simulink model "gps_time_integrator_test"  (R2016b)
settings: Solver=VariableStepAuto  StartTime=0.0  StopTime=6000  RelTol=1e-3
values from neighbouring files (symbols this model uses):
  fsw_params = init_fsw_params()    [GPS_processing_test_init.m]
libraries: gps x1, GPS_processing_lib x1, GPS_time_lib x1, time_conversion_lib x1, MET_lib x1, time_coord_rotation_lib x1, tle2eci_coarse_lib x1
settings Model: Creator=taylorreynolds  LastModifiedBy=taylorreynolds

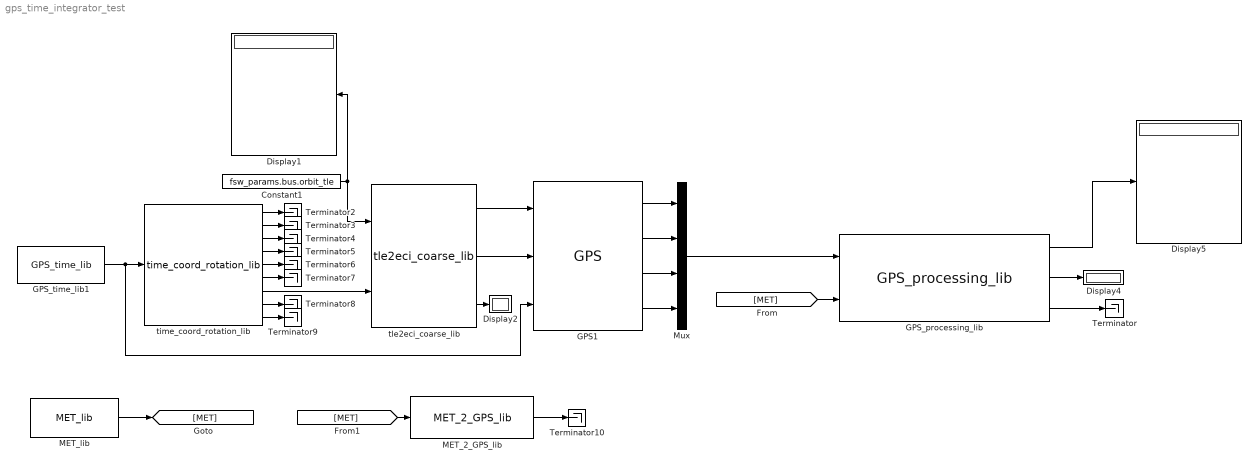
== system gps_time_integrator_test ==
  Constant1 : Constant  Value=fsw_params.bus.orbit_tle
  Display{1..2,4..5} (4 alike) : Display
  GPS1 : gps/GPS
  GPS_processing_lib : GPS_processing_lib/GPS_processing_lib
  GPS_time_lib1 : GPS_time_lib/GPS_time_lib
  MET_2_GPS_lib : time_conversion_lib/MET_2_GPS_lib
  MET_lib : MET_lib/MET_lib
  Mux : Mux  Inputs=[3 3 2 1]
  Terminator{,2..10} (10 alike) : Terminator
  time_coord_rotation_lib : time_coord_rotation_lib/time_coord_rotation_lib
  tle2eci_coarse_lib : tle2eci_coarse_lib/tle2eci_coarse_lib
  wires:
  GPS1/1 -> Mux/1
  GPS1/2 -> Mux/2
  GPS1/4 -> Mux/4
  Mux/1 -> GPS_processing_lib/1
  Constant1/1 -> Display1/1, tle2eci_coarse_lib/1
  GPS1/3 -> Mux/3
  tle2eci_coarse_lib/1 -> GPS1/1
  tle2eci_coarse_lib/2 -> GPS1/2
  GPS_processing_lib/3 -> Terminator/1
  tle2eci_coarse_lib/3 -> Display2/1
  GPS_processing_lib/2 -> Display4/1
  time_coord_rotation_lib/7 -> tle2eci_coarse_lib/2
  GPS_processing_lib/1 -> Display5/1
  time_coord_rotation_lib/1 -> Terminator2/1
  time_coord_rotation_lib/2 -> Terminator3/1
  time_coord_rotation_lib/3 -> Terminator4/1
  time_coord_rotation_lib/4 -> Terminator5/1
  time_coord_rotation_lib/5 -> Terminator6/1
  time_coord_rotation_lib/6 -> Terminator7/1
  time_coord_rotation_lib/8 -> Terminator8/1
  time_coord_rotation_lib/9 -> Terminator9/1
  MET_lib/1 -> [MET]
  [MET] -> GPS_processing_lib/2
  [MET] -> MET_2_GPS_lib/1
  MET_2_GPS_lib/1 -> Terminator10/1
  GPS_time_lib1/1 -> GPS1/3, time_coord_rotation_lib/1
